simulink library "ammclib_bam_S32K3xx"  (R2016a)
settings: Solver=VariableStepAuto  SolverMode=SingleTasking  StartTime=0.0  StopTime=10.0  RelTol=1e-3
undefined symbols (not defined in the file or in its folder): a1, a2, ADCMaxError, autoCalcEn, b0, b1, b2, cfg, dgain, escale, f16A1, f16A2, f16ADCMaxError, f16B0, f16B1, f16B2, f16C1, f16CC1sc, f16CC1sc_D, f16CC1sc_Q, f16CC2sc, f16CC2sc_D, f16CC2sc_Q, f16DerivGain, f16EGain, f16FiltCoef, f16HystOff, f16HystOn, f16IGain, f16IntegGain, f16IntegGain_D, f16IntegGain_Q, f16IntegGainQ, f16Kd, f16KLs, f16Kq, f16KRs, f16Limit, f16LowerLimit, f16LowerLimit_D, f16LowerLimit_Q, f16LowerLimitQ, f16ModIndex, f16OutValOff, f16OutValOn, f16PropGain, f16PropGain_D, f16PropGain_Q, f16PropGainQ, f16RampDown, f16RampUp, f16UGain, f16UpperLimit, f16UpperLimit_D, f16UpperLimit_Q, f16UpperLimitQ, f16WIGain, f32A1, f32A2, f32ADCMaxError ... (+180)
(part 50 of 50)

== system ammclib_bam_S32K3xx/GFLIB/F32/GFLIB_Atan_F32/copyright ==

== system ammclib_bam_S32K3xx/GFLIB/F32/GFLIB_Atan_F32/copyright2 ==

== system ammclib_bam_S32K3xx/GFLIB/F32/GFLIB_ControllerPIDpAW_F32/copyright ==

== system ammclib_bam_S32K3xx/GFLIB/F32/GFLIB_ControllerPIDpAW_F32/copyright2 ==

== system ammclib_bam_S32K3xx/GFLIB/F32/GFLIB_ControllerPIpAW_F32/copyright ==

== system ammclib_bam_S32K3xx/GFLIB/F32/GFLIB_ControllerPIpAW_F32/copyright2 ==

== system ammclib_bam_S32K3xx/GFLIB/F32/GFLIB_ControllerPIp_F32/copyright ==

== system ammclib_bam_S32K3xx/GFLIB/F32/GFLIB_ControllerPIp_F32/copyright2 ==

== system ammclib_bam_S32K3xx/GFLIB/F32/GFLIB_ControllerPIrAW_F32/copyright ==

== system ammclib_bam_S32K3xx/GFLIB/F32/GFLIB_ControllerPIrAW_F32/copyright2 ==

== system ammclib_bam_S32K3xx/GFLIB/F32/GFLIB_ControllerPIr_F32/copyright ==

== system ammclib_bam_S32K3xx/GFLIB/F32/GFLIB_ControllerPIr_F32/copyright2 ==

== system ammclib_bam_S32K3xx/GFLIB/F32/GFLIB_Cos_F32/copyright ==

== system ammclib_bam_S32K3xx/GFLIB/F32/GFLIB_Cos_F32/copyright2 ==

== system ammclib_bam_S32K3xx/GFLIB/F32/GFLIB_Hyst_F32/copyright ==

== system ammclib_bam_S32K3xx/GFLIB/F32/GFLIB_Hyst_F32/copyright2 ==

== system ammclib_bam_S32K3xx/GFLIB/F32/GFLIB_IntegratorTR_F32/copyright ==

== system ammclib_bam_S32K3xx/GFLIB/F32/GFLIB_IntegratorTR_F32/copyright2 ==

== system ammclib_bam_S32K3xx/GFLIB/F32/GFLIB_Limit_F32/copyright ==

== system ammclib_bam_S32K3xx/GFLIB/F32/GFLIB_Limit_F32/copyright2 ==

== system ammclib_bam_S32K3xx/GFLIB/F32/GFLIB_LowerLimit_F32/copyright ==

== system ammclib_bam_S32K3xx/GFLIB/F32/GFLIB_LowerLimit_F32/copyright2 ==

== system ammclib_bam_S32K3xx/GFLIB/F32/GFLIB_Lut1D_F32/copyright ==

== system ammclib_bam_S32K3xx/GFLIB/F32/GFLIB_Lut1D_F32/copyright2 ==

== system ammclib_bam_S32K3xx/GFLIB/F32/GFLIB_Lut2D_F32/copyright ==

== system ammclib_bam_S32K3xx/GFLIB/F32/GFLIB_Lut2D_F32/copyright2 ==

== system ammclib_bam_S32K3xx/GFLIB/F32/GFLIB_Ramp_F32/copyright ==

== system ammclib_bam_S32K3xx/GFLIB/F32/GFLIB_Ramp_F32/copyright2 ==

== system ammclib_bam_S32K3xx/GFLIB/F32/GFLIB_Sign_F32/copyright ==

== system ammclib_bam_S32K3xx/GFLIB/F32/GFLIB_Sign_F32/copyright2 ==

== system ammclib_bam_S32K3xx/GFLIB/F32/GFLIB_SinCos_F32/copyright ==

== system ammclib_bam_S32K3xx/GFLIB/F32/GFLIB_SinCos_F32/copyright2 ==

== system ammclib_bam_S32K3xx/GFLIB/F32/GFLIB_Sin_F32/copyright ==

== system ammclib_bam_S32K3xx/GFLIB/F32/GFLIB_Sin_F32/copyright2 ==

== system ammclib_bam_S32K3xx/GFLIB/F32/GFLIB_Sqrt_F32/copyright ==

== system ammclib_bam_S32K3xx/GFLIB/F32/GFLIB_Sqrt_F32/copyright2 ==

== system ammclib_bam_S32K3xx/GFLIB/F32/GFLIB_Tan_F32/copyright ==

== system ammclib_bam_S32K3xx/GFLIB/F32/GFLIB_Tan_F32/copyright2 ==

== system ammclib_bam_S32K3xx/GFLIB/F32/GFLIB_UpperLimit_F32/copyright ==

== system ammclib_bam_S32K3xx/GFLIB/F32/GFLIB_UpperLimit_F32/copyright2 ==

== system ammclib_bam_S32K3xx/GFLIB/F32/GFLIB_VMin_F32/copyright ==

== system ammclib_bam_S32K3xx/GFLIB/F32/GFLIB_VMin_F32/copyright2 ==

== system ammclib_bam_S32K3xx/GFLIB/F32/GFLIB_VectorLimit_F32/copyright ==

== system ammclib_bam_S32K3xx/GFLIB/F32/GFLIB_VectorLimit_F32/copyright2 ==

== system ammclib_bam_S32K3xx/GFLIB/FLT/GFLIB_Acos_FLT/copyright ==

== system ammclib_bam_S32K3xx/GFLIB/FLT/GFLIB_Acos_FLT/copyright2 ==

== system ammclib_bam_S32K3xx/GFLIB/FLT/GFLIB_Asin_FLT/copyright ==

== system ammclib_bam_S32K3xx/GFLIB/FLT/GFLIB_Asin_FLT/copyright2 ==

== system ammclib_bam_S32K3xx/GFLIB/FLT/GFLIB_AtanYXShifted_FLT/copyright ==

== system ammclib_bam_S32K3xx/GFLIB/FLT/GFLIB_AtanYXShifted_FLT/copyright2 ==

== system ammclib_bam_S32K3xx/GFLIB/FLT/GFLIB_AtanYX_FLT/copyright ==

== system ammclib_bam_S32K3xx/GFLIB/FLT/GFLIB_AtanYX_FLT/copyright2 ==

== system ammclib_bam_S32K3xx/GFLIB/FLT/GFLIB_Atan_FLT/copyright ==

== system ammclib_bam_S32K3xx/GFLIB/FLT/GFLIB_Atan_FLT/copyright2 ==

== system ammclib_bam_S32K3xx/GFLIB/FLT/GFLIB_ControllerPIDpAW_FLT/copyright ==

== system ammclib_bam_S32K3xx/GFLIB/FLT/GFLIB_ControllerPIDpAW_FLT/copyright2 ==

== system ammclib_bam_S32K3xx/GFLIB/FLT/GFLIB_ControllerPIpAW_FLT/copyright ==

== system ammclib_bam_S32K3xx/GFLIB/FLT/GFLIB_ControllerPIpAW_FLT/copyright2 ==

== system ammclib_bam_S32K3xx/GFLIB/FLT/GFLIB_ControllerPIp_FLT/copyright ==

== system ammclib_bam_S32K3xx/GFLIB/FLT/GFLIB_ControllerPIp_FLT/copyright2 ==

== system ammclib_bam_S32K3xx/GFLIB/FLT/GFLIB_ControllerPIrAW_FLT/copyright ==

== system ammclib_bam_S32K3xx/GFLIB/FLT/GFLIB_ControllerPIrAW_FLT/copyright2 ==

== system ammclib_bam_S32K3xx/GFLIB/FLT/GFLIB_ControllerPIr_FLT/copyright ==

== system ammclib_bam_S32K3xx/GFLIB/FLT/GFLIB_ControllerPIr_FLT/copyright2 ==

== system ammclib_bam_S32K3xx/GFLIB/FLT/GFLIB_Cos_FLT/copyright ==

== system ammclib_bam_S32K3xx/GFLIB/FLT/GFLIB_Cos_FLT/copyright2 ==

== system ammclib_bam_S32K3xx/GFLIB/FLT/GFLIB_Hyst_FLT/copyright ==

== system ammclib_bam_S32K3xx/GFLIB/FLT/GFLIB_Hyst_FLT/copyright2 ==

== system ammclib_bam_S32K3xx/GFLIB/FLT/GFLIB_IntegratorTR_FLT/copyright ==

== system ammclib_bam_S32K3xx/GFLIB/FLT/GFLIB_IntegratorTR_FLT/copyright2 ==

== system ammclib_bam_S32K3xx/GFLIB/FLT/GFLIB_Limit_FLT/copyright ==

== system ammclib_bam_S32K3xx/GFLIB/FLT/GFLIB_Limit_FLT/copyright2 ==

== system ammclib_bam_S32K3xx/GFLIB/FLT/GFLIB_Log10_FLT/copyright ==

== system ammclib_bam_S32K3xx/GFLIB/FLT/GFLIB_Log10_FLT/copyright2 ==

== system ammclib_bam_S32K3xx/GFLIB/FLT/GFLIB_LowerLimit_FLT/copyright ==

== system ammclib_bam_S32K3xx/GFLIB/FLT/GFLIB_LowerLimit_FLT/copyright2 ==

== system ammclib_bam_S32K3xx/GFLIB/FLT/GFLIB_Lut1D_FLT/copyright ==

== system ammclib_bam_S32K3xx/GFLIB/FLT/GFLIB_Lut1D_FLT/copyright2 ==

== system ammclib_bam_S32K3xx/GFLIB/FLT/GFLIB_Lut2D_FLT/copyright ==

== system ammclib_bam_S32K3xx/GFLIB/FLT/GFLIB_Lut2D_FLT/copyright2 ==

== system ammclib_bam_S32K3xx/GFLIB/FLT/GFLIB_Ramp_FLT/copyright ==

== system ammclib_bam_S32K3xx/GFLIB/FLT/GFLIB_Ramp_FLT/copyright2 ==

== system ammclib_bam_S32K3xx/GFLIB/FLT/GFLIB_Sign_FLT/copyright ==

== system ammclib_bam_S32K3xx/GFLIB/FLT/GFLIB_Sign_FLT/copyright2 ==

== system ammclib_bam_S32K3xx/GFLIB/FLT/GFLIB_SinCos_FLT/copyright ==

== system ammclib_bam_S32K3xx/GFLIB/FLT/GFLIB_SinCos_FLT/copyright2 ==

== system ammclib_bam_S32K3xx/GFLIB/FLT/GFLIB_Sin_FLT/copyright ==

== system ammclib_bam_S32K3xx/GFLIB/FLT/GFLIB_Sin_FLT/copyright2 ==

== system ammclib_bam_S32K3xx/GFLIB/FLT/GFLIB_Sqrt_FLT/copyright ==

== system ammclib_bam_S32K3xx/GFLIB/FLT/GFLIB_Sqrt_FLT/copyright2 ==

== system ammclib_bam_S32K3xx/GFLIB/FLT/GFLIB_Tan_FLT/copyright ==

== system ammclib_bam_S32K3xx/GFLIB/FLT/GFLIB_Tan_FLT/copyright2 ==

== system ammclib_bam_S32K3xx/GFLIB/FLT/GFLIB_UpperLimit_FLT/copyright ==

== system ammclib_bam_S32K3xx/GFLIB/FLT/GFLIB_UpperLimit_FLT/copyright2 ==

== system ammclib_bam_S32K3xx/GFLIB/FLT/GFLIB_VLog10_FLT/copyright ==

== system ammclib_bam_S32K3xx/GFLIB/FLT/GFLIB_VLog10_FLT/copyright2 ==

== system ammclib_bam_S32K3xx/GFLIB/FLT/GFLIB_VMin_FLT/copyright ==

== system ammclib_bam_S32K3xx/GFLIB/FLT/GFLIB_VMin_FLT/copyright2 ==

== system ammclib_bam_S32K3xx/GFLIB/FLT/GFLIB_VectorLimit_FLT/copyright ==

== system ammclib_bam_S32K3xx/GFLIB/FLT/GFLIB_VectorLimit_FLT/copyright2 ==

== system ammclib_bam_S32K3xx/GMCLIB/F16/GMCLIB_BetaProjection3Ph_F16/copyright ==

== system ammclib_bam_S32K3xx/GMCLIB/F16/GMCLIB_BetaProjection3Ph_F16/copyright2 ==

== system ammclib_bam_S32K3xx/GMCLIB/F16/GMCLIB_BetaProjection_F16/copyright ==

== system ammclib_bam_S32K3xx/GMCLIB/F16/GMCLIB_BetaProjection_F16/copyright2 ==

== system ammclib_bam_S32K3xx/GMCLIB/F16/GMCLIB_Clark6Ph_F16/copyright ==

== system ammclib_bam_S32K3xx/GMCLIB/F16/GMCLIB_Clark6Ph_F16/copyright2 ==

== system ammclib_bam_S32K3xx/GMCLIB/F16/GMCLIB_ClarkInv6Ph_F16/copyright ==

== system ammclib_bam_S32K3xx/GMCLIB/F16/GMCLIB_ClarkInv6Ph_F16/copyright2 ==

== system ammclib_bam_S32K3xx/GMCLIB/F16/GMCLIB_ClarkInv_F16/copyright ==

== system ammclib_bam_S32K3xx/GMCLIB/F16/GMCLIB_ClarkInv_F16/copyright2 ==

== system ammclib_bam_S32K3xx/GMCLIB/F16/GMCLIB_Clark_F16/copyright ==

== system ammclib_bam_S32K3xx/GMCLIB/F16/GMCLIB_Clark_F16/copyright2 ==

== system ammclib_bam_S32K3xx/GMCLIB/F16/GMCLIB_DecouplingPMSM_F16/copyright ==

== system ammclib_bam_S32K3xx/GMCLIB/F16/GMCLIB_DecouplingPMSM_F16/copyright2 ==

== system ammclib_bam_S32K3xx/GMCLIB/F16/GMCLIB_DoubleSwitching_F16/copyright ==

== system ammclib_bam_S32K3xx/GMCLIB/F16/GMCLIB_DoubleSwitching_F16/copyright2 ==

== system ammclib_bam_S32K3xx/GMCLIB/F16/GMCLIB_ElimDcBusRip_F16/copyright ==

== system ammclib_bam_S32K3xx/GMCLIB/F16/GMCLIB_ElimDcBusRip_F16/copyright2 ==

== system ammclib_bam_S32K3xx/GMCLIB/F16/GMCLIB_ParkInv_F16/copyright ==

== system ammclib_bam_S32K3xx/GMCLIB/F16/GMCLIB_ParkInv_F16/copyright2 ==

== system ammclib_bam_S32K3xx/GMCLIB/F16/GMCLIB_Park_F16/copyright ==

== system ammclib_bam_S32K3xx/GMCLIB/F16/GMCLIB_Park_F16/copyright2 ==

== system ammclib_bam_S32K3xx/GMCLIB/F16/GMCLIB_PwmIct_F16/copyright ==

== system ammclib_bam_S32K3xx/GMCLIB/F16/GMCLIB_PwmIct_F16/copyright2 ==

== system ammclib_bam_S32K3xx/GMCLIB/F16/GMCLIB_SvmSci_F16/copyright ==

== system ammclib_bam_S32K3xx/GMCLIB/F16/GMCLIB_SvmSci_F16/copyright2 ==

== system ammclib_bam_S32K3xx/GMCLIB/F16/GMCLIB_SvmStd6Ph_F16/copyright ==

== system ammclib_bam_S32K3xx/GMCLIB/F16/GMCLIB_SvmStd6Ph_F16/copyright2 ==

== system ammclib_bam_S32K3xx/GMCLIB/F16/GMCLIB_SvmStd_F16/copyright ==

== system ammclib_bam_S32K3xx/GMCLIB/F16/GMCLIB_SvmStd_F16/copyright2 ==

== system ammclib_bam_S32K3xx/GMCLIB/F16/GMCLIB_SvmU0n_F16/copyright ==

== system ammclib_bam_S32K3xx/GMCLIB/F16/GMCLIB_SvmU0n_F16/copyright2 ==

== system ammclib_bam_S32K3xx/GMCLIB/F16/GMCLIB_SvmU7n_F16/copyright ==

== system ammclib_bam_S32K3xx/GMCLIB/F16/GMCLIB_SvmU7n_F16/copyright2 ==

== system ammclib_bam_S32K3xx/GMCLIB/F16/GMCLIB_VRot_F16/copyright ==

== system ammclib_bam_S32K3xx/GMCLIB/F16/GMCLIB_VRot_F16/copyright2 ==

== system ammclib_bam_S32K3xx/GMCLIB/F16/GMCLIB_VUnit_F16/copyright ==

== system ammclib_bam_S32K3xx/GMCLIB/F16/GMCLIB_VUnit_F16/copyright2 ==

== system ammclib_bam_S32K3xx/GMCLIB/F16/GMCLIB_Vmag2coord_F16/copyright ==

== system ammclib_bam_S32K3xx/GMCLIB/F16/GMCLIB_Vmag2coord_F16/copyright2 ==

== system ammclib_bam_S32K3xx/GMCLIB/F16/GMCLIB_Vpol2xy_F16/copyright ==

== system ammclib_bam_S32K3xx/GMCLIB/F16/GMCLIB_Vpol2xy_F16/copyright2 ==

== system ammclib_bam_S32K3xx/GMCLIB/F16/GMCLIB_Vxy2pol_F16/copyright ==

== system ammclib_bam_S32K3xx/GMCLIB/F16/GMCLIB_Vxy2pol_F16/copyright2 ==

== system ammclib_bam_S32K3xx/GMCLIB/F32/GMCLIB_BetaProjection3Ph_F32/copyright ==

== system ammclib_bam_S32K3xx/GMCLIB/F32/GMCLIB_BetaProjection3Ph_F32/copyright2 ==

== system ammclib_bam_S32K3xx/GMCLIB/F32/GMCLIB_BetaProjection_F32/copyright ==

== system ammclib_bam_S32K3xx/GMCLIB/F32/GMCLIB_BetaProjection_F32/copyright2 ==

== system ammclib_bam_S32K3xx/GMCLIB/F32/GMCLIB_Clark6Ph_F32/copyright ==

== system ammclib_bam_S32K3xx/GMCLIB/F32/GMCLIB_Clark6Ph_F32/copyright2 ==

== system ammclib_bam_S32K3xx/GMCLIB/F32/GMCLIB_ClarkInv6Ph_F32/copyright ==

== system ammclib_bam_S32K3xx/GMCLIB/F32/GMCLIB_ClarkInv6Ph_F32/copyright2 ==

== system ammclib_bam_S32K3xx/GMCLIB/F32/GMCLIB_ClarkInv_F32/copyright ==

== system ammclib_bam_S32K3xx/GMCLIB/F32/GMCLIB_ClarkInv_F32/copyright2 ==

== system ammclib_bam_S32K3xx/GMCLIB/F32/GMCLIB_Clark_F32/copyright ==

== system ammclib_bam_S32K3xx/GMCLIB/F32/GMCLIB_Clark_F32/copyright2 ==

== system ammclib_bam_S32K3xx/GMCLIB/F32/GMCLIB_DecouplingPMSM_F32/copyright ==

== system ammclib_bam_S32K3xx/GMCLIB/F32/GMCLIB_DecouplingPMSM_F32/copyright2 ==

== system ammclib_bam_S32K3xx/GMCLIB/F32/GMCLIB_ElimDcBusRip_F32/copyright ==

== system ammclib_bam_S32K3xx/GMCLIB/F32/GMCLIB_ElimDcBusRip_F32/copyright2 ==

== system ammclib_bam_S32K3xx/GMCLIB/F32/GMCLIB_ParkInv_F32/copyright ==

== system ammclib_bam_S32K3xx/GMCLIB/F32/GMCLIB_ParkInv_F32/copyright2 ==

== system ammclib_bam_S32K3xx/GMCLIB/F32/GMCLIB_Park_F32/copyright ==

== system ammclib_bam_S32K3xx/GMCLIB/F32/GMCLIB_Park_F32/copyright2 ==

== system ammclib_bam_S32K3xx/GMCLIB/F32/GMCLIB_PwmIct_F32/copyright ==

== system ammclib_bam_S32K3xx/GMCLIB/F32/GMCLIB_PwmIct_F32/copyright2 ==

== system ammclib_bam_S32K3xx/GMCLIB/F32/GMCLIB_SvmSci_F32/copyright ==

== system ammclib_bam_S32K3xx/GMCLIB/F32/GMCLIB_SvmSci_F32/copyright2 ==

== system ammclib_bam_S32K3xx/GMCLIB/F32/GMCLIB_SvmStd6Ph_F32/copyright ==

== system ammclib_bam_S32K3xx/GMCLIB/F32/GMCLIB_SvmStd6Ph_F32/copyright2 ==

== system ammclib_bam_S32K3xx/GMCLIB/F32/GMCLIB_SvmStd_F32/copyright ==

== system ammclib_bam_S32K3xx/GMCLIB/F32/GMCLIB_SvmStd_F32/copyright2 ==

== system ammclib_bam_S32K3xx/GMCLIB/F32/GMCLIB_SvmU0n_F32/copyright ==

== system ammclib_bam_S32K3xx/GMCLIB/F32/GMCLIB_SvmU0n_F32/copyright2 ==

== system ammclib_bam_S32K3xx/GMCLIB/F32/GMCLIB_SvmU7n_F32/copyright ==

== system ammclib_bam_S32K3xx/GMCLIB/F32/GMCLIB_SvmU7n_F32/copyright2 ==

== system ammclib_bam_S32K3xx/GMCLIB/F32/GMCLIB_VRot_F32/copyright ==

== system ammclib_bam_S32K3xx/GMCLIB/F32/GMCLIB_VRot_F32/copyright2 ==

== system ammclib_bam_S32K3xx/GMCLIB/F32/GMCLIB_VUnit_F32/copyright ==

== system ammclib_bam_S32K3xx/GMCLIB/F32/GMCLIB_VUnit_F32/copyright2 ==

== system ammclib_bam_S32K3xx/GMCLIB/F32/GMCLIB_Vmag2coord_F32/copyright ==

== system ammclib_bam_S32K3xx/GMCLIB/F32/GMCLIB_Vmag2coord_F32/copyright2 ==

== system ammclib_bam_S32K3xx/GMCLIB/F32/GMCLIB_Vpol2xy_F32/copyright ==

== system ammclib_bam_S32K3xx/GMCLIB/F32/GMCLIB_Vpol2xy_F32/copyright2 ==

== system ammclib_bam_S32K3xx/GMCLIB/F32/GMCLIB_Vxy2pol_F32/copyright ==

== system ammclib_bam_S32K3xx/GMCLIB/F32/GMCLIB_Vxy2pol_F32/copyright2 ==

== system ammclib_bam_S32K3xx/GMCLIB/FLT/GMCLIB_BetaProjection3Ph_FLT/copyright ==

== system ammclib_bam_S32K3xx/GMCLIB/FLT/GMCLIB_BetaProjection3Ph_FLT/copyright2 ==

== system ammclib_bam_S32K3xx/GMCLIB/FLT/GMCLIB_BetaProjection_FLT/copyright ==

== system ammclib_bam_S32K3xx/GMCLIB/FLT/GMCLIB_BetaProjection_FLT/copyright2 ==

== system ammclib_bam_S32K3xx/GMCLIB/FLT/GMCLIB_Clark6Ph_FLT/copyright ==

== system ammclib_bam_S32K3xx/GMCLIB/FLT/GMCLIB_Clark6Ph_FLT/copyright2 ==

== system ammclib_bam_S32K3xx/GMCLIB/FLT/GMCLIB_ClarkInv6Ph_FLT/copyright ==

== system ammclib_bam_S32K3xx/GMCLIB/FLT/GMCLIB_ClarkInv6Ph_FLT/copyright2 ==

== system ammclib_bam_S32K3xx/GMCLIB/FLT/GMCLIB_ClarkInv_FLT/copyright ==

== system ammclib_bam_S32K3xx/GMCLIB/FLT/GMCLIB_ClarkInv_FLT/copyright2 ==

== system ammclib_bam_S32K3xx/GMCLIB/FLT/GMCLIB_Clark_FLT/copyright ==

== system ammclib_bam_S32K3xx/GMCLIB/FLT/GMCLIB_Clark_FLT/copyright2 ==

== system ammclib_bam_S32K3xx/GMCLIB/FLT/GMCLIB_DecouplingPMSM_FLT/copyright ==

== system ammclib_bam_S32K3xx/GMCLIB/FLT/GMCLIB_DecouplingPMSM_FLT/copyright2 ==

== system ammclib_bam_S32K3xx/GMCLIB/FLT/GMCLIB_ElimDcBusRip_FLT/copyright ==

== system ammclib_bam_S32K3xx/GMCLIB/FLT/GMCLIB_ElimDcBusRip_FLT/copyright2 ==

== system ammclib_bam_S32K3xx/GMCLIB/FLT/GMCLIB_ParkInv_FLT/copyright ==

== system ammclib_bam_S32K3xx/GMCLIB/FLT/GMCLIB_ParkInv_FLT/copyright2 ==

== system ammclib_bam_S32K3xx/GMCLIB/FLT/GMCLIB_Park_FLT/copyright ==

== system ammclib_bam_S32K3xx/GMCLIB/FLT/GMCLIB_Park_FLT/copyright2 ==

== system ammclib_bam_S32K3xx/GMCLIB/FLT/GMCLIB_PwmIct_FLT/copyright ==

== system ammclib_bam_S32K3xx/GMCLIB/FLT/GMCLIB_PwmIct_FLT/copyright2 ==

== system ammclib_bam_S32K3xx/GMCLIB/FLT/GMCLIB_SvmSci_FLT/copyright ==

== system ammclib_bam_S32K3xx/GMCLIB/FLT/GMCLIB_SvmSci_FLT/copyright2 ==

== system ammclib_bam_S32K3xx/GMCLIB/FLT/GMCLIB_SvmStd6Ph_FLT/copyright ==

== system ammclib_bam_S32K3xx/GMCLIB/FLT/GMCLIB_SvmStd6Ph_FLT/copyright2 ==

== system ammclib_bam_S32K3xx/GMCLIB/FLT/GMCLIB_SvmStd_FLT/copyright ==

== system ammclib_bam_S32K3xx/GMCLIB/FLT/GMCLIB_SvmStd_FLT/copyright2 ==

== system ammclib_bam_S32K3xx/GMCLIB/FLT/GMCLIB_SvmU0n_FLT/copyright ==

== system ammclib_bam_S32K3xx/GMCLIB/FLT/GMCLIB_SvmU0n_FLT/copyright2 ==

== system ammclib_bam_S32K3xx/GMCLIB/FLT/GMCLIB_SvmU7n_FLT/copyright ==

== system ammclib_bam_S32K3xx/GMCLIB/FLT/GMCLIB_SvmU7n_FLT/copyright2 ==

== system ammclib_bam_S32K3xx/GMCLIB/FLT/GMCLIB_VRot_FLT/copyright ==

== system ammclib_bam_S32K3xx/GMCLIB/FLT/GMCLIB_VRot_FLT/copyright2 ==

== system ammclib_bam_S32K3xx/GMCLIB/FLT/GMCLIB_VUnit_FLT/copyright ==

== system ammclib_bam_S32K3xx/GMCLIB/FLT/GMCLIB_VUnit_FLT/copyright2 ==

== system ammclib_bam_S32K3xx/GMCLIB/FLT/GMCLIB_Vmag2coord_FLT/copyright ==

== system ammclib_bam_S32K3xx/GMCLIB/FLT/GMCLIB_Vmag2coord_FLT/copyright2 ==

== system ammclib_bam_S32K3xx/GMCLIB/FLT/GMCLIB_Vpol2xy_FLT/copyright ==

== system ammclib_bam_S32K3xx/GMCLIB/FLT/GMCLIB_Vpol2xy_FLT/copyright2 ==

== system ammclib_bam_S32K3xx/GMCLIB/FLT/GMCLIB_Vxy2pol_FLT/copyright ==

== system ammclib_bam_S32K3xx/GMCLIB/FLT/GMCLIB_Vxy2pol_FLT/copyright2 ==

== system ammclib_bam_S32K3xx/GMCLIB/Generic/GMCLIB_SpreadPWM/copyright ==

== system ammclib_bam_S32K3xx/GMCLIB/Generic/GMCLIB_SpreadPWM/copyright2 ==

== system ammclib_bam_S32K3xx/MLIB/F16/MLIB_AbsSat_F16/copyright ==

== system ammclib_bam_S32K3xx/MLIB/F16/MLIB_AbsSat_F16/copyright2 ==

== system ammclib_bam_S32K3xx/MLIB/F16/MLIB_Abs_F16/copyright ==

== system ammclib_bam_S32K3xx/MLIB/F16/MLIB_Abs_F16/copyright2 ==

== system ammclib_bam_S32K3xx/MLIB/F16/MLIB_AddSat_F16/copyright ==

== system ammclib_bam_S32K3xx/MLIB/F16/MLIB_AddSat_F16/copyright2 ==

== system ammclib_bam_S32K3xx/MLIB/F16/MLIB_Add_F16/copyright ==

== system ammclib_bam_S32K3xx/MLIB/F16/MLIB_Add_F16/copyright2 ==

== system ammclib_bam_S32K3xx/MLIB/F16/MLIB_ConvertPU_F16F32/copyright ==

== system ammclib_bam_S32K3xx/MLIB/F16/MLIB_ConvertPU_F16F32/copyright2 ==

== system ammclib_bam_S32K3xx/MLIB/F16/MLIB_ConvertPU_F16FLT/copyright ==

== system ammclib_bam_S32K3xx/MLIB/F16/MLIB_ConvertPU_F16FLT/copyright2 ==

== system ammclib_bam_S32K3xx/MLIB/F16/MLIB_Convert_F16F32/copyright ==

== system ammclib_bam_S32K3xx/MLIB/F16/MLIB_Convert_F16F32/copyright2 ==

== system ammclib_bam_S32K3xx/MLIB/F16/MLIB_Convert_F16FLT/copyright ==

== system ammclib_bam_S32K3xx/MLIB/F16/MLIB_Convert_F16FLT/copyright2 ==

== system ammclib_bam_S32K3xx/MLIB/F16/MLIB_DivSat_F16/copyright ==

== system ammclib_bam_S32K3xx/MLIB/F16/MLIB_DivSat_F16/copyright2 ==

== system ammclib_bam_S32K3xx/MLIB/F16/MLIB_Div_F16/copyright ==

== system ammclib_bam_S32K3xx/MLIB/F16/MLIB_Div_F16/copyright2 ==

== system ammclib_bam_S32K3xx/MLIB/F16/MLIB_MacSat_F16/copyright ==

== system ammclib_bam_S32K3xx/MLIB/F16/MLIB_MacSat_F16/copyright2 ==

== system ammclib_bam_S32K3xx/MLIB/F16/MLIB_Mac_F16/copyright ==

== system ammclib_bam_S32K3xx/MLIB/F16/MLIB_Mac_F16/copyright2 ==

== system ammclib_bam_S32K3xx/MLIB/F16/MLIB_Mnac_F16/copyright ==

== system ammclib_bam_S32K3xx/MLIB/F16/MLIB_Mnac_F16/copyright2 ==

== system ammclib_bam_S32K3xx/MLIB/F16/MLIB_Msu_F16/copyright ==

== system ammclib_bam_S32K3xx/MLIB/F16/MLIB_Msu_F16/copyright2 ==

== system ammclib_bam_S32K3xx/MLIB/F16/MLIB_MulSat_F16/copyright ==

== system ammclib_bam_S32K3xx/MLIB/F16/MLIB_MulSat_F16/copyright2 ==

== system ammclib_bam_S32K3xx/MLIB/F16/MLIB_Mul_F16/copyright ==

== system ammclib_bam_S32K3xx/MLIB/F16/MLIB_Mul_F16/copyright2 ==

== system ammclib_bam_S32K3xx/MLIB/F16/MLIB_NegSat_F16/copyright ==

== system ammclib_bam_S32K3xx/MLIB/F16/MLIB_NegSat_F16/copyright2 ==

== system ammclib_bam_S32K3xx/MLIB/F16/MLIB_Neg_F16/copyright ==

== system ammclib_bam_S32K3xx/MLIB/F16/MLIB_Neg_F16/copyright2 ==

== system ammclib_bam_S32K3xx/MLIB/F16/MLIB_Norm_F16/copyright ==

== system ammclib_bam_S32K3xx/MLIB/F16/MLIB_Norm_F16/copyright2 ==

== system ammclib_bam_S32K3xx/MLIB/F16/MLIB_RndSat_F16F32/copyright ==

== system ammclib_bam_S32K3xx/MLIB/F16/MLIB_RndSat_F16F32/copyright2 ==

== system ammclib_bam_S32K3xx/MLIB/F16/MLIB_Round_F16/copyright ==

== system ammclib_bam_S32K3xx/MLIB/F16/MLIB_Round_F16/copyright2 ==

== system ammclib_bam_S32K3xx/MLIB/F16/MLIB_ShBiSat_F16/copyright ==

== system ammclib_bam_S32K3xx/MLIB/F16/MLIB_ShBiSat_F16/copyright2 ==

== system ammclib_bam_S32K3xx/MLIB/F16/MLIB_ShBi_F16/copyright ==

== system ammclib_bam_S32K3xx/MLIB/F16/MLIB_ShBi_F16/copyright2 ==

== system ammclib_bam_S32K3xx/MLIB/F16/MLIB_ShLSat_F16/copyright ==

== system ammclib_bam_S32K3xx/MLIB/F16/MLIB_ShLSat_F16/copyright2 ==

== system ammclib_bam_S32K3xx/MLIB/F16/MLIB_ShL_F16/copyright ==

== system ammclib_bam_S32K3xx/MLIB/F16/MLIB_ShL_F16/copyright2 ==

== system ammclib_bam_S32K3xx/MLIB/F16/MLIB_ShR_F16/copyright ==

== system ammclib_bam_S32K3xx/MLIB/F16/MLIB_ShR_F16/copyright2 ==

== system ammclib_bam_S32K3xx/MLIB/F16/MLIB_SubSat_F16/copyright ==

== system ammclib_bam_S32K3xx/MLIB/F16/MLIB_SubSat_F16/copyright2 ==

== system ammclib_bam_S32K3xx/MLIB/F16/MLIB_Sub_F16/copyright ==

== system ammclib_bam_S32K3xx/MLIB/F16/MLIB_Sub_F16/copyright2 ==

== system ammclib_bam_S32K3xx/MLIB/F16/MLIB_VAdd_F16/copyright ==

== system ammclib_bam_S32K3xx/MLIB/F16/MLIB_VAdd_F16/copyright2 ==

== system ammclib_bam_S32K3xx/MLIB/F16/MLIB_VMac_F16/copyright ==

== system ammclib_bam_S32K3xx/MLIB/F16/MLIB_VMac_F16/copyright2 ==

== system ammclib_bam_S32K3xx/MLIB/F16/MLIB_VScale_F16/copyright ==

== system ammclib_bam_S32K3xx/MLIB/F16/MLIB_VScale_F16/copyright2 ==

== system ammclib_bam_S32K3xx/MLIB/F16/MLIB_VSub_F16/copyright ==

== system ammclib_bam_S32K3xx/MLIB/F16/MLIB_VSub_F16/copyright2 ==

== system ammclib_bam_S32K3xx/MLIB/F32/MLIB_AbsSat_F32/copyright ==

== system ammclib_bam_S32K3xx/MLIB/F32/MLIB_AbsSat_F32/copyright2 ==

== system ammclib_bam_S32K3xx/MLIB/F32/MLIB_Abs_F32/copyright ==

== system ammclib_bam_S32K3xx/MLIB/F32/MLIB_Abs_F32/copyright2 ==

== system ammclib_bam_S32K3xx/MLIB/F32/MLIB_AddSat_F32/copyright ==

== system ammclib_bam_S32K3xx/MLIB/F32/MLIB_AddSat_F32/copyright2 ==

== system ammclib_bam_S32K3xx/MLIB/F32/MLIB_Add_F32/copyright ==

== system ammclib_bam_S32K3xx/MLIB/F32/MLIB_Add_F32/copyright2 ==

== system ammclib_bam_S32K3xx/MLIB/F32/MLIB_ConvertPU_F32F16/copyright ==

== system ammclib_bam_S32K3xx/MLIB/F32/MLIB_ConvertPU_F32F16/copyright2 ==

== system ammclib_bam_S32K3xx/MLIB/F32/MLIB_ConvertPU_F32FLT/copyright ==

== system ammclib_bam_S32K3xx/MLIB/F32/MLIB_ConvertPU_F32FLT/copyright2 ==

== system ammclib_bam_S32K3xx/MLIB/F32/MLIB_Convert_F32F16/copyright ==

== system ammclib_bam_S32K3xx/MLIB/F32/MLIB_Convert_F32F16/copyright2 ==

== system ammclib_bam_S32K3xx/MLIB/F32/MLIB_Convert_F32FLT/copyright ==

== system ammclib_bam_S32K3xx/MLIB/F32/MLIB_Convert_F32FLT/copyright2 ==

== system ammclib_bam_S32K3xx/MLIB/F32/MLIB_DivSatAccurate_F32/copyright ==

== system ammclib_bam_S32K3xx/MLIB/F32/MLIB_DivSatAccurate_F32/copyright2 ==

== system ammclib_bam_S32K3xx/MLIB/F32/MLIB_DivSat_F32/copyright ==

== system ammclib_bam_S32K3xx/MLIB/F32/MLIB_DivSat_F32/copyright2 ==

== system ammclib_bam_S32K3xx/MLIB/F32/MLIB_Div_F32/copyright ==

== system ammclib_bam_S32K3xx/MLIB/F32/MLIB_Div_F32/copyright2 ==

== system ammclib_bam_S32K3xx/MLIB/F32/MLIB_MacSat_F32/copyright ==

== system ammclib_bam_S32K3xx/MLIB/F32/MLIB_MacSat_F32/copyright2 ==

== system ammclib_bam_S32K3xx/MLIB/F32/MLIB_Mac_F32/copyright ==

== system ammclib_bam_S32K3xx/MLIB/F32/MLIB_Mac_F32/copyright2 ==

== system ammclib_bam_S32K3xx/MLIB/F32/MLIB_Mnac_F32/copyright ==

== system ammclib_bam_S32K3xx/MLIB/F32/MLIB_Mnac_F32/copyright2 ==

== system ammclib_bam_S32K3xx/MLIB/F32/MLIB_Msu_F32/copyright ==

== system ammclib_bam_S32K3xx/MLIB/F32/MLIB_Msu_F32/copyright2 ==

== system ammclib_bam_S32K3xx/MLIB/F32/MLIB_MulSat_F32/copyright ==

== system ammclib_bam_S32K3xx/MLIB/F32/MLIB_MulSat_F32/copyright2 ==

== system ammclib_bam_S32K3xx/MLIB/F32/MLIB_Mul_F32/copyright ==

== system ammclib_bam_S32K3xx/MLIB/F32/MLIB_Mul_F32/copyright2 ==

== system ammclib_bam_S32K3xx/MLIB/F32/MLIB_NegSat_F32/copyright ==

== system ammclib_bam_S32K3xx/MLIB/F32/MLIB_NegSat_F32/copyright2 ==

== system ammclib_bam_S32K3xx/MLIB/F32/MLIB_Neg_F32/copyright ==

== system ammclib_bam_S32K3xx/MLIB/F32/MLIB_Neg_F32/copyright2 ==

== system ammclib_bam_S32K3xx/MLIB/F32/MLIB_Norm_F32/copyright ==

== system ammclib_bam_S32K3xx/MLIB/F32/MLIB_Norm_F32/copyright2 ==

== system ammclib_bam_S32K3xx/MLIB/F32/MLIB_Round_F32/copyright ==

== system ammclib_bam_S32K3xx/MLIB/F32/MLIB_Round_F32/copyright2 ==

== system ammclib_bam_S32K3xx/MLIB/F32/MLIB_ShBiSat_F32/copyright ==

== system ammclib_bam_S32K3xx/MLIB/F32/MLIB_ShBiSat_F32/copyright2 ==

== system ammclib_bam_S32K3xx/MLIB/F32/MLIB_ShBi_F32/copyright ==

== system ammclib_bam_S32K3xx/MLIB/F32/MLIB_ShBi_F32/copyright2 ==

== system ammclib_bam_S32K3xx/MLIB/F32/MLIB_ShLSat_F32/copyright ==

== system ammclib_bam_S32K3xx/MLIB/F32/MLIB_ShLSat_F32/copyright2 ==

== system ammclib_bam_S32K3xx/MLIB/F32/MLIB_ShL_F32/copyright ==

== system ammclib_bam_S32K3xx/MLIB/F32/MLIB_ShL_F32/copyright2 ==

== system ammclib_bam_S32K3xx/MLIB/F32/MLIB_ShR_F32/copyright ==

== system ammclib_bam_S32K3xx/MLIB/F32/MLIB_ShR_F32/copyright2 ==

== system ammclib_bam_S32K3xx/MLIB/F32/MLIB_SubSat_F32/copyright ==

== system ammclib_bam_S32K3xx/MLIB/F32/MLIB_SubSat_F32/copyright2 ==

== system ammclib_bam_S32K3xx/MLIB/F32/MLIB_Sub_F32/copyright ==

== system ammclib_bam_S32K3xx/MLIB/F32/MLIB_Sub_F32/copyright2 ==

== system ammclib_bam_S32K3xx/MLIB/F32/MLIB_VAdd_F32/copyright ==

== system ammclib_bam_S32K3xx/MLIB/F32/MLIB_VAdd_F32/copyright2 ==

== system ammclib_bam_S32K3xx/MLIB/F32/MLIB_VMac_F32/copyright ==

== system ammclib_bam_S32K3xx/MLIB/F32/MLIB_VMac_F32/copyright2 ==

== system ammclib_bam_S32K3xx/MLIB/F32/MLIB_VScale_F32/copyright ==

== system ammclib_bam_S32K3xx/MLIB/F32/MLIB_VScale_F32/copyright2 ==

== system ammclib_bam_S32K3xx/MLIB/F32/MLIB_VSub_F32/copyright ==

== system ammclib_bam_S32K3xx/MLIB/F32/MLIB_VSub_F32/copyright2 ==

== system ammclib_bam_S32K3xx/MLIB/F32F16F16/MLIB_MacSat_F32F16F16/copyright ==

== system ammclib_bam_S32K3xx/MLIB/F32F16F16/MLIB_MacSat_F32F16F16/copyright2 ==

== system ammclib_bam_S32K3xx/MLIB/F32F16F16/MLIB_Mac_F32F16F16/copyright ==

== system ammclib_bam_S32K3xx/MLIB/F32F16F16/MLIB_Mac_F32F16F16/copyright2 ==

== system ammclib_bam_S32K3xx/MLIB/F32F16F16/MLIB_Mnac_F32F16F16/copyright ==

== system ammclib_bam_S32K3xx/MLIB/F32F16F16/MLIB_Mnac_F32F16F16/copyright2 ==

== system ammclib_bam_S32K3xx/MLIB/F32F16F16/MLIB_Msu_F32F16F16/copyright ==

== system ammclib_bam_S32K3xx/MLIB/F32F16F16/MLIB_Msu_F32F16F16/copyright2 ==

== system ammclib_bam_S32K3xx/MLIB/F32F16F16/MLIB_MulSat_F32F16F16/copyright ==

== system ammclib_bam_S32K3xx/MLIB/F32F16F16/MLIB_MulSat_F32F16F16/copyright2 ==

== system ammclib_bam_S32K3xx/MLIB/F32F16F16/MLIB_Mul_F32F16F16/copyright ==

== system ammclib_bam_S32K3xx/MLIB/F32F16F16/MLIB_Mul_F32F16F16/copyright2 ==

== system ammclib_bam_S32K3xx/MLIB/F32F16F16/MLIB_VMac_F32F16F16/copyright ==

== system ammclib_bam_S32K3xx/MLIB/F32F16F16/MLIB_VMac_F32F16F16/copyright2 ==

== system ammclib_bam_S32K3xx/MLIB/FLT/MLIB_Abs_FLT/copyright ==

== system ammclib_bam_S32K3xx/MLIB/FLT/MLIB_Abs_FLT/copyright2 ==

== system ammclib_bam_S32K3xx/MLIB/FLT/MLIB_Add_FLT/copyright ==

== system ammclib_bam_S32K3xx/MLIB/FLT/MLIB_Add_FLT/copyright2 ==

== system ammclib_bam_S32K3xx/MLIB/FLT/MLIB_ConvertPU_FLTF16/copyright ==

== system ammclib_bam_S32K3xx/MLIB/FLT/MLIB_ConvertPU_FLTF16/copyright2 ==

== system ammclib_bam_S32K3xx/MLIB/FLT/MLIB_ConvertPU_FLTF32/copyright ==

== system ammclib_bam_S32K3xx/MLIB/FLT/MLIB_ConvertPU_FLTF32/copyright2 ==

== system ammclib_bam_S32K3xx/MLIB/FLT/MLIB_Convert_FLTF16/copyright ==

== system ammclib_bam_S32K3xx/MLIB/FLT/MLIB_Convert_FLTF16/copyright2 ==

== system ammclib_bam_S32K3xx/MLIB/FLT/MLIB_Convert_FLTF32/copyright ==

== system ammclib_bam_S32K3xx/MLIB/FLT/MLIB_Convert_FLTF32/copyright2 ==

== system ammclib_bam_S32K3xx/MLIB/FLT/MLIB_Div_FLT/copyright ==

== system ammclib_bam_S32K3xx/MLIB/FLT/MLIB_Div_FLT/copyright2 ==

== system ammclib_bam_S32K3xx/MLIB/FLT/MLIB_Mac_FLT/copyright ==

== system ammclib_bam_S32K3xx/MLIB/FLT/MLIB_Mac_FLT/copyright2 ==

== system ammclib_bam_S32K3xx/MLIB/FLT/MLIB_Mnac_FLT/copyright ==

== system ammclib_bam_S32K3xx/MLIB/FLT/MLIB_Mnac_FLT/copyright2 ==

== system ammclib_bam_S32K3xx/MLIB/FLT/MLIB_Msu_FLT/copyright ==

== system ammclib_bam_S32K3xx/MLIB/FLT/MLIB_Msu_FLT/copyright2 ==

== system ammclib_bam_S32K3xx/MLIB/FLT/MLIB_Mul_FLT/copyright ==

== system ammclib_bam_S32K3xx/MLIB/FLT/MLIB_Mul_FLT/copyright2 ==

== system ammclib_bam_S32K3xx/MLIB/FLT/MLIB_Neg_FLT/copyright ==

== system ammclib_bam_S32K3xx/MLIB/FLT/MLIB_Neg_FLT/copyright2 ==

== system ammclib_bam_S32K3xx/MLIB/FLT/MLIB_Sub_FLT/copyright ==

== system ammclib_bam_S32K3xx/MLIB/FLT/MLIB_Sub_FLT/copyright2 ==

== system ammclib_bam_S32K3xx/MLIB/FLT/MLIB_VAdd_FLT/copyright ==

== system ammclib_bam_S32K3xx/MLIB/FLT/MLIB_VAdd_FLT/copyright2 ==

== system ammclib_bam_S32K3xx/MLIB/FLT/MLIB_VMac_FLT/copyright ==

== system ammclib_bam_S32K3xx/MLIB/FLT/MLIB_VMac_FLT/copyright2 ==

== system ammclib_bam_S32K3xx/MLIB/FLT/MLIB_VScale_FLT/copyright ==

== system ammclib_bam_S32K3xx/MLIB/FLT/MLIB_VScale_FLT/copyright2 ==

== system ammclib_bam_S32K3xx/MLIB/FLT/MLIB_VSub_FLT/copyright ==

== system ammclib_bam_S32K3xx/MLIB/FLT/MLIB_VSub_FLT/copyright2 ==
